simulink model "Exercise24"  (R2017a)
settings: Solver=VariableStepAuto  StartTime=0.0  StopTime=50  MaxStep=0.002  RelTol=1e-3
undefined symbols (not defined in the file): Freq, k, Tau
settings Model: Creator=JakobLab  LastModifiedBy=JakobLab

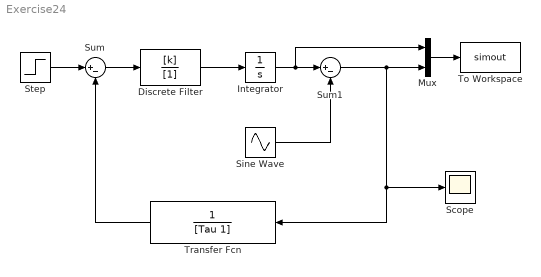
== system Exercise24 ==
  Discrete Filter : DiscreteFilter  Numerator=[k]  Denominator=[1]  SampleTime=1
  Integrator : Integrator
  Mux : Mux  Inputs=2
  Scope : Scope
  Sine Wave : Sin  Frequency=Freq  Phase=pi/2  SampleTime=0
  Step : Step  SampleTime=0
  Sum : Sum  Inputs=|+-
  Sum1 : Sum  Inputs=|+-
  To Workspace : ToWorkspace  VariableName=simout  SaveFormat=Structure With Time  SampleTime=-1
  Transfer Fcn : TransferFcn  Denominator=[Tau 1]
  wires:
  Mux/1 -> To Workspace/1
  Sine Wave/1 -> Sum1/2
  Sum1/1 -> Transfer Fcn/1, Scope/1, Mux/2
  Step/1 -> Sum/1
  Sum/1 -> Discrete Filter/1
  Discrete Filter/1 -> Integrator/1
  Integrator/1 -> Mux/1, Sum1/1
  Transfer Fcn/1 -> Sum/2
